simulink model "simulacao"  (R2015b)
settings: Solver=ode45  StartTime=0.0  StopTime=10.0  RelTol=1e-3
settings Model: Creator=Davi  LastModifiedBy=Moises
settings DataIOCC: SaveFormat=Array
settings HardwareCC: ProdBitPerPointer=32  ProdLargestAtomicFloat=None  ProdIntDivRoundTo=Undefined  ProdEndianess=Unspecified  ProdWordSize=32  ProdHWDeviceType=32-bit Generic
settings GRTTargetCC: GeneratePreprocessorConditionals=Disable all
settings ConfigComp: CovModelRefEnable=Off

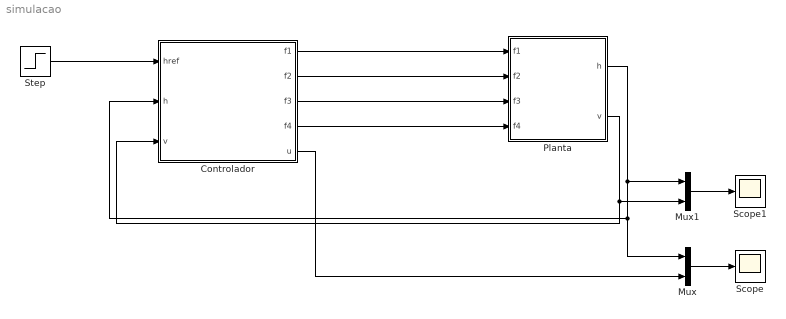
== system simulacao ==
  Controlador : Subsystem  mask{Kp=5, Kd=2, m=1, g=9.81}
  Mux : Mux  Inputs=2
  Mux1 : Mux  Inputs=2
  Planta : Subsystem  mask{m=1, g=9.81}
      mask prompts: m "massa"; g "gravidade"
  Scope : Scope
  Scope1 : Scope
  Step : Step  SampleTime=0
  wires:
  Controlador/1(f1) -> Planta/1(f1)
  Controlador/2(f2) -> Planta/2(f2)
  Controlador/3(f3) -> Planta/3(f3)
  Controlador/4(f4) -> Planta/4(f4)
  Controlador/5(u) -> Mux/2
  Mux/1 -> Scope/1
  Step/1 -> Controlador/1(href)
  Planta/1(h) -> Mux1/1, Controlador/2(h), Mux/1
  Planta/2("v ") -> Mux1/2, Controlador/3(v)
  Mux1/1 -> Scope1/1

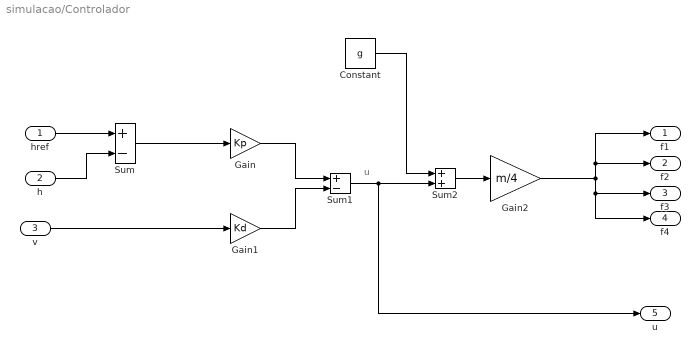
== system simulacao/Controlador ==
  note: u
  href : Inport
  h : Inport  Port=2
  v : Inport  Port=3
  Constant : Constant  Value=g
  Gain : Gain  Gain=Kp
  Gain1 : Gain  Gain=Kd
  Gain2 : Gain  Gain=m/4
  Sum : Sum  Inputs=+-
  Sum1 : Sum  Inputs=+-
  Sum2 : Sum
  f1 : Outport
  f2 : Outport  Port=2
  f3 : Outport  Port=3
  f4 : Outport  Port=4
  u : Outport  Port=5
  wires:
  h/1 -> Sum/2
  Gain/1 -> Sum1/1
  Sum/1 -> Gain/1
  href/1 -> Sum/1
  v/1 -> Gain1/1
  Gain1/1 -> Sum1/2
  Sum1/1 -> u/1, Sum2/2
  Constant/1 -> Sum2/1
  Sum2/1 -> Gain2/1
  Gain2/1 -> f3/1, f4/1, f2/1, f1/1

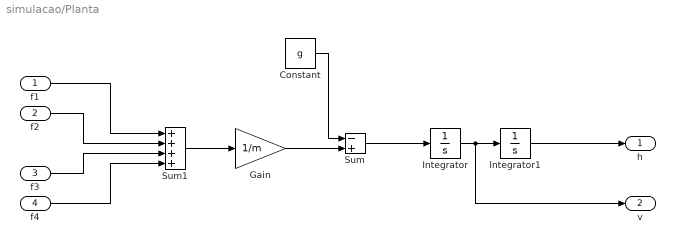
== system simulacao/Planta ==
  f1 : Inport
  f2 : Inport  Port=2
  f3 : Inport  Port=3
  f4 : Inport  Port=4
  Constant : Constant  Value=g
  Gain : Gain  Gain=1/m
  Integrator : Integrator
  Integrator1 : Integrator
  Sum : Sum  Inputs=-+
  Sum1 : Sum  Inputs=++++
  h : Outport
  "v " : Outport  Port=2
  wires:
  f3/1 -> Sum1/3
  Gain/1 -> Sum/2
  Integrator/1 -> "v "/1, Integrator1/1
  Constant/1 -> Sum/1
  Integrator1/1 -> h/1
  f2/1 -> Sum1/2
  Sum/1 -> Integrator/1
  Sum1/1 -> Gain/1
  f4/1 -> Sum1/4
  f1/1 -> Sum1/1
